simulink model "MCR2_Example_Gazebo_Publisher_Subscriber"  (R2024a)
settings: Solver=VariableStepAuto  StartTime=0.0  StopTime=30  RelTol=1e-3
undefined symbols (not defined in the file): Angular, Linear
libraries: robotlib x4, robotgazebolib x1
settings Model: Creator=mario  LastModifiedBy=mario

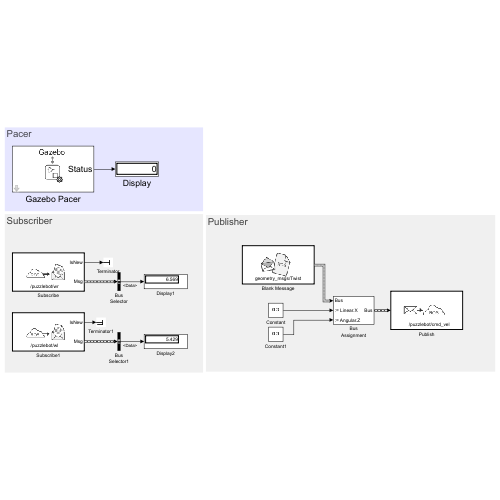
[thumbnail: Simulink's stored preview of the top-level diagram]
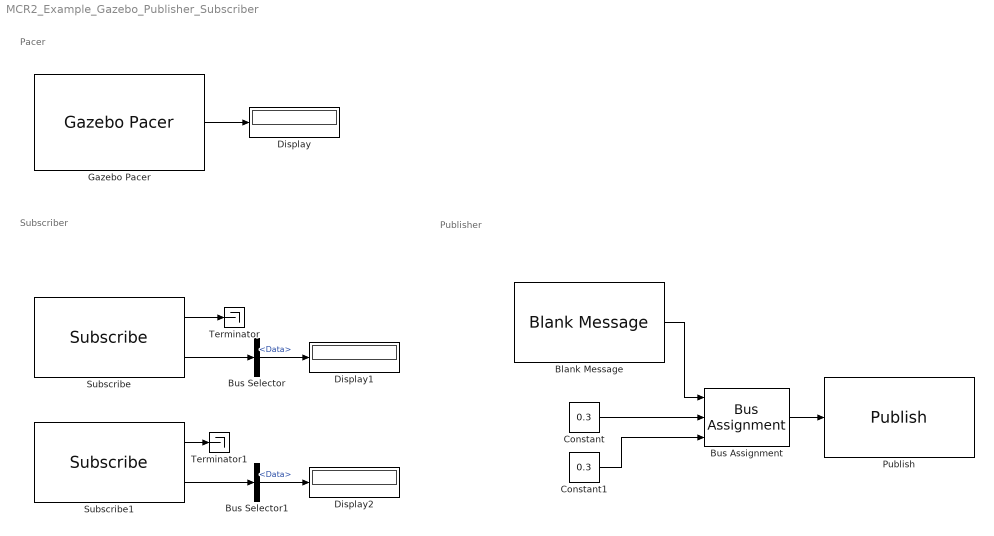
== system MCR2_Example_Gazebo_Publisher_Subscriber ==
  note: Publisher
  note: Subscriber
  note: Pacer
  Blank Message : robotlib/Blank Message  messageClass=Message  entityType=geometry_msgs/Twist  messageType=geometry_msgs/Twist  SampleTime=0.01  legacyBusStruct=off
  Bus Assignment : BusAssignment  AssignedSignals=Linear.X,Angular.Z
  Bus Selector : BusSelector  OutputSignals=Data
  Bus Selector1 : BusSelector  OutputSignals=Data
  Constant : Constant  Value=0.3  SampleTime=0.01
  Constant1 : Constant  Value=0.3  SampleTime=0.01
  Display : Display
  Display1 : Display
  Display2 : Display
  Gazebo Pacer : robotgazebolib/Gazebo Pacer  ResetBehavior=Reset Gazebo simulation time and scene  SampleTime=0.001
  Publish : robotlib/Publish  topicSource=Select from ROS network  topic=/puzzlebot/cmd_vel  messageType=geometry_msgs/Twist  legacyBusStruct=off  messageQueueLength=1
  Subscribe : robotlib/Subscribe  topicSource=Select from ROS network  topic=/puzzlebot/wr  messageType=std_msgs/Float32  SampleTime=0.010  legacyBusStruct=off  messageQueueLength=1
  Subscribe1 : robotlib/Subscribe  topicSource=Select from ROS network  topic=/puzzlebot/wl  messageType=std_msgs/Float32  SampleTime=0.01  legacyBusStruct=off  messageQueueLength=1
  Terminator : Terminator
  Terminator1 : Terminator
  wires:
  Gazebo Pacer/1 -> Display/1
  Subscribe/2 -> Bus Selector/1
  Subscribe/1 -> Terminator/1
  Subscribe1/1 -> Terminator1/1
  Subscribe1/2 -> Bus Selector1/1
  Bus Selector/1 -> Display1/1  "<Data>"
  Bus Selector1/1 -> Display2/1  "<Data>"
  Bus Assignment/1 -> Publish/1
  Blank Message/1 -> Bus Assignment/1
  Constant/1 -> Bus Assignment/2
  Constant1/1 -> Bus Assignment/3
